simulink library "circulationForce_ul"  (R2018b)
settings: Solver=VariableStepAuto  StartTime=0.0  StopTime=10.0  RelTol=1e-3
undefined symbols (not defined in the file): A, cd, oceanPeriod, rho, vsquared, xOn, zOn
settings Model: Creator=Erin B  LastModifiedBy=mcobb

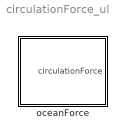
== system circulationForce_ul ==
  oceanForce : Subsystem

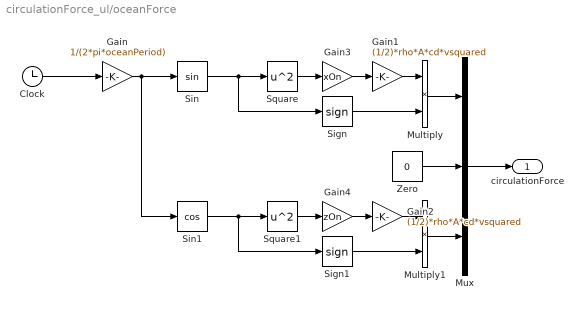
== system circulationForce_ul/oceanForce ==
  Clock : Clock
  Gain : Gain  Gain=1/(2*pi*oceanPeriod)
  Gain1 : Gain  Gain=(1/2)*rho*A*cd*vsquared
  Gain2 : Gain  Gain=(1/2)*rho*A*cd*vsquared
  Gain3 : Gain  Gain=xOn
  Gain4 : Gain  Gain=zOn
  Multiply : Product
  Multiply1 : Product
  Mux : Mux  Inputs=3
  Sign : Signum
  Sign1 : Signum
  Sin : Trigonometry
  Sin1 : Trigonometry  Operator=cos
  Square : Math  Operator=square  SaturateOnIntegerOverflow=on
  Square1 : Math  Operator=square  SaturateOnIntegerOverflow=on
  Zero : Constant  Value=0  OutDataTypeStr=Inherit: Inherit via back propagation
  circulationForce : Outport
  wires:
  Sin/1 -> Sign/1, Square/1
  Clock/1 -> Gain/1
  Gain/1 -> Sin1/1, Sin/1
  Square/1 -> Gain3/1
  Gain1/1 -> Multiply/1
  Multiply/1 -> Mux/1
  Sign/1 -> Multiply/2
  Sin1/1 -> Square1/1, Sign1/1
  Sign1/1 -> Multiply1/2
  Multiply1/1 -> Mux/3
  Gain2/1 -> Multiply1/1
  Square1/1 -> Gain4/1
  Zero/1 -> Mux/2
  Mux/1 -> circulationForce/1
  Gain3/1 -> Gain1/1
  Gain4/1 -> Gain2/1
